simulink model "SMARTFARM_PROJ"  (R2013b)
settings: Solver=ode3  SolverMode=SingleTasking  StartTime=0.0  StopTime=10.0  RelTol=1e-3
PreLoadFcn:
  | waijung.modelPreload; % Required for working with Waijung Blockset. Do not remove.
undefined symbols (not defined in the file): HSEOSC, Link, LQFP176, ST, STM32F417IG
libraries: stm32f4_io_lib x6, stm32f4_adc_lib x1, stm32f4_device_config_lib x1
(part 2 of 2)

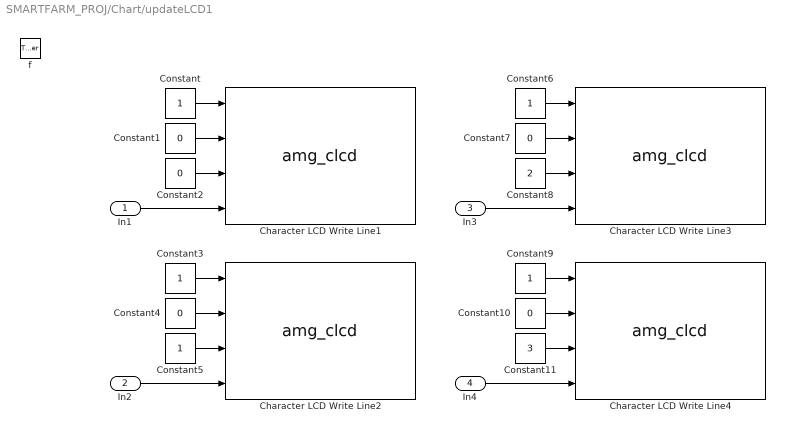
== system SMARTFARM_PROJ/Chart/updateLCD1 ==
  In1 : Inport  OutDataTypeStr=uint8  PortDimensions=[1 16]
  In2 : Inport  Port=2  OutDataTypeStr=uint8  PortDimensions=[1 16]
  In3 : Inport  Port=3  OutDataTypeStr=uint8  PortDimensions=[1 16]
  In4 : Inport  Port=4  OutDataTypeStr=uint8  PortDimensions=[1 16]
  f : TriggerPort  TriggerType=function-call
      settings: CopyFcn=Stateflow.SLINSF.SimulinkMan.removeBlockPreDeleteFcn  PreDeleteFcn=Stateflow.SLINSF.SimulinkMan.unsafePredeleteFcn
  Character LCD Write Line1 : S-Function  FunctionName=amg_clcd  Parameters=module,configuration,inputtypearray,outputtypearray,confstr,sampletime,sampletimestr,blockid  EnableBusSupport=off  mask(amg_clcd){configuration=Transaction, module=1, model=amg CLCD Std, interface=4-bits, linecount=4, columncount=20, gpiotype=Push-pull, controlport=E, control_rs=15, control_rw=13, control_en=11, dataport=A, data0=7, data1=5, data2=3, data3=1, usestringbuffer=off, stringbuffer=<empty>, varname=, inputtypearray=[4 -1 -1 -1 -1], outputtypearray=[0], confstr=["4","4","20","PP","E","15","11","13","","A","","","","","7","5","3","1","0","","1","0","0","0","1","0","0","0","0","stm32f4"], sampletime=-1, sampletimestr=-1, blockid=ChartupdateLCD1CharacterLCDWriteLine1}
      mask prompts: model "LCD model:"; linecount "Number of lines:"; columncount "Number of columns:"; gpiotype "GPIO Output type:"; controlport "GPIO control port:"; control_rs "GPIO control pin, RS:"; control_rw "GPIO control pin, RW:"; control_en "GPIO control pin, EN:"; dataport "GPIO data D[7:4] port"; data0 "GPIO data pin, D4:"; data1 "GPIO data pin, D5:"; data2 "GPIO data pin, D6:"; data3 "GPIO data pin, D7:"; usestringbuffer "Use string buffer"; stringbuffer "String buffer"; varname "Variable name"; inputtypearray "Input type array"; outputtypearray "Output type array"; confstr "Configuration string"; sampletime "Sample time (sec)"; sampletimestr "Compiled sample time (sec) in string"
      mask help:
      | Note for cmd:
      | 1 - Clear specified LCD line display before write data to LCD.
      | Otherwise (e.g. 0) - Write data without clearing LCD Line.
      |
      | Position:
      | x = 0, First Character (from left to right)
      | y = 0, Top Line
      mask init:
      | amg_clcd_callback('init');
      mask Help: web(fullfile(waijungdocroot,'amg_clcd_write.htm'), '-browser')
      mask TypeOptions configuration: Setup | Transaction
      mask Callback configuration: amg_clcd_callback('configuration');
      mask TypeOptions module: 1 | 2 | 3 | 4
      mask TypeOptions model: amg CLCD Std
      mask TypeOptions interface: 4-bits
      mask TypeOptions gpiotype: Push-pull | Open-drain
      mask TypeOptions controlport: A | B | C | D | E | F | G | H | I
      mask TypeOptions control_rs: 0 | 1 | 2 | 3 | 4 | 5 | 6 | 7 | 8 | 9 | 10 | 11 | 12 | 13 | 14 | 15
      mask TypeOptions control_rw: 0 | 1 | 2 | 3 | 4 | 5 | 6 | 7 | 8 | 9 | 10 | 11 | 12 | 13 | 14 | 15
      mask TypeOptions control_en: 0 | 1 | 2 | 3 | 4 | 5 | 6 | 7 | 8 | 9 | 10 | 11 | 12 | 13 | 14 | 15
      mask TypeOptions dataport: A | B | C | D | E | F | G | H | I
      mask TypeOptions data0: 0 | 1 | 2 | 3 | 4 | 5 | 6 | 7 | 8 | 9 | 10 | 11 | 12 | 13 | 14 | 15
      mask TypeOptions data1: 0 | 1 | 2 | 3 | 4 | 5 | 6 | 7 | 8 | 9 | 10 | 11 | 12 | 13 | 14 | 15
      mask TypeOptions data2: 0 | 1 | 2 | 3 | 4 | 5 | 6 | 7 | 8 | 9 | 10 | 11 | 12 | 13 | 14 | 15
      mask TypeOptions data3: 0 | 1 | 2 | 3 | 4 | 5 | 6 | 7 | 8 | 9 | 10 | 11 | 12 | 13 | 14 | 15
      mask Callback usestringbuffer: amg_clcd_callback('usestringbuffer');
      mask TypeOptions stringbuffer: <empty>
      mask Callback varname: amg_clcd_callback('varname');
      mask Callback confstr: amg_clcd_callback('confstr');
      mask Callback sampletime: amg_clcd_callback('sampletime');
      mask Callback sampletimestr: amg_clcd_callback('sampletimestr');
      mask Callback blockid: amg_clcd_callback('blockid');
      mask Display: text(0.5, 0.5, 'Module: CLCD1 (Write)\nTs (sec): -1','ver','middle','hor','center');port_label('input', 1,'cmd');port_label('input', 2,'xpos');port_label('input', 3,'ypos');port_label('input', 4,'str');
  Character LCD Write Line2 : S-Function  FunctionName=amg_clcd  Parameters=module,configuration,inputtypearray,outputtypearray,confstr,sampletime,sampletimestr,blockid  EnableBusSupport=off  mask(amg_clcd){configuration=Transaction, module=1, model=amg CLCD Std, interface=4-bits, linecount=4, columncount=20, gpiotype=Push-pull, controlport=E, control_rs=15, control_rw=13, control_en=11, dataport=A, data0=7, data1=5, data2=3, data3=1, usestringbuffer=off, stringbuffer=<empty>, varname=, inputtypearray=[4 -1 -1 -1 -1], outputtypearray=[0], confstr=["4","4","20","PP","E","15","11","13","","A","","","","","7","5","3","1","0","","1","0","0","0","1","0","0","0","0","stm32f4"], sampletime=-1, sampletimestr=-1, blockid=ChartupdateLCD1CharacterLCDWriteLine2}
      mask prompts: model "LCD model:"; linecount "Number of lines:"; columncount "Number of columns:"; gpiotype "GPIO Output type:"; controlport "GPIO control port:"; control_rs "GPIO control pin, RS:"; control_rw "GPIO control pin, RW:"; control_en "GPIO control pin, EN:"; dataport "GPIO data D[7:4] port"; data0 "GPIO data pin, D4:"; data1 "GPIO data pin, D5:"; data2 "GPIO data pin, D6:"; data3 "GPIO data pin, D7:"; usestringbuffer "Use string buffer"; stringbuffer "String buffer"; varname "Variable name"; inputtypearray "Input type array"; outputtypearray "Output type array"; confstr "Configuration string"; sampletime "Sample time (sec)"; sampletimestr "Compiled sample time (sec) in string"
      mask help:
      | Note for cmd:
      | 1 - Clear specified LCD line display before write data to LCD.
      | Otherwise (e.g. 0) - Write data without clearing LCD Line.
      |
      | Position:
      | x = 0, First Character (from left to right)
      | y = 0, Top Line
      mask init:
      | amg_clcd_callback('init');
      mask Help: web(fullfile(waijungdocroot,'amg_clcd_write.htm'), '-browser')
      mask TypeOptions configuration: Setup | Transaction
      mask Callback configuration: amg_clcd_callback('configuration');
      mask TypeOptions module: 1 | 2 | 3 | 4
      mask TypeOptions model: amg CLCD Std
      mask TypeOptions interface: 4-bits
      mask TypeOptions gpiotype: Push-pull | Open-drain
      mask TypeOptions controlport: A | B | C | D | E | F | G | H | I
      mask TypeOptions control_rs: 0 | 1 | 2 | 3 | 4 | 5 | 6 | 7 | 8 | 9 | 10 | 11 | 12 | 13 | 14 | 15
      mask TypeOptions control_rw: 0 | 1 | 2 | 3 | 4 | 5 | 6 | 7 | 8 | 9 | 10 | 11 | 12 | 13 | 14 | 15
      mask TypeOptions control_en: 0 | 1 | 2 | 3 | 4 | 5 | 6 | 7 | 8 | 9 | 10 | 11 | 12 | 13 | 14 | 15
      mask TypeOptions dataport: A | B | C | D | E | F | G | H | I
      mask TypeOptions data0: 0 | 1 | 2 | 3 | 4 | 5 | 6 | 7 | 8 | 9 | 10 | 11 | 12 | 13 | 14 | 15
      mask TypeOptions data1: 0 | 1 | 2 | 3 | 4 | 5 | 6 | 7 | 8 | 9 | 10 | 11 | 12 | 13 | 14 | 15
      mask TypeOptions data2: 0 | 1 | 2 | 3 | 4 | 5 | 6 | 7 | 8 | 9 | 10 | 11 | 12 | 13 | 14 | 15
      mask TypeOptions data3: 0 | 1 | 2 | 3 | 4 | 5 | 6 | 7 | 8 | 9 | 10 | 11 | 12 | 13 | 14 | 15
      mask Callback usestringbuffer: amg_clcd_callback('usestringbuffer');
      mask TypeOptions stringbuffer: <empty>
      mask Callback varname: amg_clcd_callback('varname');
      mask Callback confstr: amg_clcd_callback('confstr');
      mask Callback sampletime: amg_clcd_callback('sampletime');
      mask Callback sampletimestr: amg_clcd_callback('sampletimestr');
      mask Callback blockid: amg_clcd_callback('blockid');
      mask Display: text(0.5, 0.5, 'Module: CLCD1 (Write)\nTs (sec): -1','ver','middle','hor','center');port_label('input', 1,'cmd');port_label('input', 2,'xpos');port_label('input', 3,'ypos');port_label('input', 4,'str');
  Character LCD Write Line3 : S-Function  FunctionName=amg_clcd  Parameters=module,configuration,inputtypearray,outputtypearray,confstr,sampletime,sampletimestr,blockid  EnableBusSupport=off  mask(amg_clcd){configuration=Transaction, module=1, model=amg CLCD Std, interface=4-bits, linecount=4, columncount=20, gpiotype=Push-pull, controlport=E, control_rs=15, control_rw=13, control_en=11, dataport=A, data0=7, data1=5, data2=3, data3=1, usestringbuffer=off, stringbuffer=<empty>, varname=, inputtypearray=[4 -1 -1 -1 -1], outputtypearray=[0], confstr=["4","4","20","PP","E","15","11","13","","A","","","","","7","5","3","1","0","","1","0","0","0","1","0","0","0","0","stm32f4"], sampletime=-1, sampletimestr=-1, blockid=ChartupdateLCD1CharacterLCDWriteLine3}
      mask prompts: model "LCD model:"; linecount "Number of lines:"; columncount "Number of columns:"; gpiotype "GPIO Output type:"; controlport "GPIO control port:"; control_rs "GPIO control pin, RS:"; control_rw "GPIO control pin, RW:"; control_en "GPIO control pin, EN:"; dataport "GPIO data D[7:4] port"; data0 "GPIO data pin, D4:"; data1 "GPIO data pin, D5:"; data2 "GPIO data pin, D6:"; data3 "GPIO data pin, D7:"; usestringbuffer "Use string buffer"; stringbuffer "String buffer"; varname "Variable name"; inputtypearray "Input type array"; outputtypearray "Output type array"; confstr "Configuration string"; sampletime "Sample time (sec)"; sampletimestr "Compiled sample time (sec) in string"
      mask help:
      | Note for cmd:
      | 1 - Clear specified LCD line display before write data to LCD.
      | Otherwise (e.g. 0) - Write data without clearing LCD Line.
      |
      | Position:
      | x = 0, First Character (from left to right)
      | y = 0, Top Line
      mask init:
      | amg_clcd_callback('init');
      mask Help: web(fullfile(waijungdocroot,'amg_clcd_write.htm'), '-browser')
      mask TypeOptions configuration: Setup | Transaction
      mask Callback configuration: amg_clcd_callback('configuration');
      mask TypeOptions module: 1 | 2 | 3 | 4
      mask TypeOptions model: amg CLCD Std
      mask TypeOptions interface: 4-bits
      mask TypeOptions gpiotype: Push-pull | Open-drain
      mask TypeOptions controlport: A | B | C | D | E | F | G | H | I
      mask TypeOptions control_rs: 0 | 1 | 2 | 3 | 4 | 5 | 6 | 7 | 8 | 9 | 10 | 11 | 12 | 13 | 14 | 15
      mask TypeOptions control_rw: 0 | 1 | 2 | 3 | 4 | 5 | 6 | 7 | 8 | 9 | 10 | 11 | 12 | 13 | 14 | 15
      mask TypeOptions control_en: 0 | 1 | 2 | 3 | 4 | 5 | 6 | 7 | 8 | 9 | 10 | 11 | 12 | 13 | 14 | 15
      mask TypeOptions dataport: A | B | C | D | E | F | G | H | I
      mask TypeOptions data0: 0 | 1 | 2 | 3 | 4 | 5 | 6 | 7 | 8 | 9 | 10 | 11 | 12 | 13 | 14 | 15
      mask TypeOptions data1: 0 | 1 | 2 | 3 | 4 | 5 | 6 | 7 | 8 | 9 | 10 | 11 | 12 | 13 | 14 | 15
      mask TypeOptions data2: 0 | 1 | 2 | 3 | 4 | 5 | 6 | 7 | 8 | 9 | 10 | 11 | 12 | 13 | 14 | 15
      mask TypeOptions data3: 0 | 1 | 2 | 3 | 4 | 5 | 6 | 7 | 8 | 9 | 10 | 11 | 12 | 13 | 14 | 15
      mask Callback usestringbuffer: amg_clcd_callback('usestringbuffer');
      mask TypeOptions stringbuffer: <empty>
      mask Callback varname: amg_clcd_callback('varname');
      mask Callback confstr: amg_clcd_callback('confstr');
      mask Callback sampletime: amg_clcd_callback('sampletime');
      mask Callback sampletimestr: amg_clcd_callback('sampletimestr');
      mask Callback blockid: amg_clcd_callback('blockid');
      mask Display: text(0.5, 0.5, 'Module: CLCD1 (Write)\nTs (sec): -1','ver','middle','hor','center');port_label('input', 1,'cmd');port_label('input', 2,'xpos');port_label('input', 3,'ypos');port_label('input', 4,'str');
  Character LCD Write Line4 : S-Function  FunctionName=amg_clcd  Parameters=module,configuration,inputtypearray,outputtypearray,confstr,sampletime,sampletimestr,blockid  EnableBusSupport=off  mask(amg_clcd){configuration=Transaction, module=1, model=amg CLCD Std, interface=4-bits, linecount=4, columncount=20, gpiotype=Push-pull, controlport=E, control_rs=15, control_rw=13, control_en=11, dataport=A, data0=7, data1=5, data2=3, data3=1, usestringbuffer=off, stringbuffer=<empty>, varname=, inputtypearray=[4 -1 -1 -1 -1], outputtypearray=[0], confstr=["4","4","20","PP","E","15","11","13","","A","","","","","7","5","3","1","0","","1","0","0","0","1","0","0","0","0","stm32f4"], sampletime=-1, sampletimestr=-1, blockid=ChartupdateLCD1CharacterLCDWriteLine4}
      mask prompts: model "LCD model:"; linecount "Number of lines:"; columncount "Number of columns:"; gpiotype "GPIO Output type:"; controlport "GPIO control port:"; control_rs "GPIO control pin, RS:"; control_rw "GPIO control pin, RW:"; control_en "GPIO control pin, EN:"; dataport "GPIO data D[7:4] port"; data0 "GPIO data pin, D4:"; data1 "GPIO data pin, D5:"; data2 "GPIO data pin, D6:"; data3 "GPIO data pin, D7:"; usestringbuffer "Use string buffer"; stringbuffer "String buffer"; varname "Variable name"; inputtypearray "Input type array"; outputtypearray "Output type array"; confstr "Configuration string"; sampletime "Sample time (sec)"; sampletimestr "Compiled sample time (sec) in string"
      mask help:
      | Note for cmd:
      | 1 - Clear specified LCD line display before write data to LCD.
      | Otherwise (e.g. 0) - Write data without clearing LCD Line.
      |
      | Position:
      | x = 0, First Character (from left to right)
      | y = 0, Top Line
      mask init:
      | amg_clcd_callback('init');
      mask Help: web(fullfile(waijungdocroot,'amg_clcd_write.htm'), '-browser')
      mask TypeOptions configuration: Setup | Transaction
      mask Callback configuration: amg_clcd_callback('configuration');
      mask TypeOptions module: 1 | 2 | 3 | 4
      mask TypeOptions model: amg CLCD Std
      mask TypeOptions interface: 4-bits
      mask TypeOptions gpiotype: Push-pull | Open-drain
      mask TypeOptions controlport: A | B | C | D | E | F | G | H | I
      mask TypeOptions control_rs: 0 | 1 | 2 | 3 | 4 | 5 | 6 | 7 | 8 | 9 | 10 | 11 | 12 | 13 | 14 | 15
      mask TypeOptions control_rw: 0 | 1 | 2 | 3 | 4 | 5 | 6 | 7 | 8 | 9 | 10 | 11 | 12 | 13 | 14 | 15
      mask TypeOptions control_en: 0 | 1 | 2 | 3 | 4 | 5 | 6 | 7 | 8 | 9 | 10 | 11 | 12 | 13 | 14 | 15
      mask TypeOptions dataport: A | B | C | D | E | F | G | H | I
      mask TypeOptions data0: 0 | 1 | 2 | 3 | 4 | 5 | 6 | 7 | 8 | 9 | 10 | 11 | 12 | 13 | 14 | 15
      mask TypeOptions data1: 0 | 1 | 2 | 3 | 4 | 5 | 6 | 7 | 8 | 9 | 10 | 11 | 12 | 13 | 14 | 15
      mask TypeOptions data2: 0 | 1 | 2 | 3 | 4 | 5 | 6 | 7 | 8 | 9 | 10 | 11 | 12 | 13 | 14 | 15
      mask TypeOptions data3: 0 | 1 | 2 | 3 | 4 | 5 | 6 | 7 | 8 | 9 | 10 | 11 | 12 | 13 | 14 | 15
      mask Callback usestringbuffer: amg_clcd_callback('usestringbuffer');
      mask TypeOptions stringbuffer: <empty>
      mask Callback varname: amg_clcd_callback('varname');
      mask Callback confstr: amg_clcd_callback('confstr');
      mask Callback sampletime: amg_clcd_callback('sampletime');
      mask Callback sampletimestr: amg_clcd_callback('sampletimestr');
      mask Callback blockid: amg_clcd_callback('blockid');
      mask Display: text(0.5, 0.5, 'Module: CLCD1 (Write)\nTs (sec): -1','ver','middle','hor','center');port_label('input', 1,'cmd');port_label('input', 2,'xpos');port_label('input', 3,'ypos');port_label('input', 4,'str');
  Constant{,3,5..6,9} (5 alike) : Constant
  Constant{1..2,4,7,10} (5 alike) : Constant  Value=0
  Constant11 : Constant  Value=3
  Constant8 : Constant  Value=2
  wires:
  In1/1 -> Character LCD Write Line1/4
  Constant/1 -> Character LCD Write Line1/1
  Constant1/1 -> Character LCD Write Line1/2
  Constant2/1 -> Character LCD Write Line1/3
  In2/1 -> Character LCD Write Line2/4
  Constant3/1 -> Character LCD Write Line2/1
  Constant4/1 -> Character LCD Write Line2/2
  Constant5/1 -> Character LCD Write Line2/3
  In3/1 -> Character LCD Write Line3/4
  Constant6/1 -> Character LCD Write Line3/1
  Constant7/1 -> Character LCD Write Line3/2
  Constant8/1 -> Character LCD Write Line3/3
  In4/1 -> Character LCD Write Line4/4
  Constant9/1 -> Character LCD Write Line4/1
  Constant10/1 -> Character LCD Write Line4/2
  Constant11/1 -> Character LCD Write Line4/3

== stateflow chart SMARTFARM_PROJ/Chart ==
  state Initialization
  state NormalOperation
    state CheckKeyPress [parallel]
      settings: executionOrder=2
      state NoKeyPressed
        en: data = 0;
      state UpKeyPressed
        en: data = 1;
        state Short
        (default) -> NormalOperation.CheckKeyPress.UpKeyPressed.Short : {UP_KEY_PRESSED;}
      state DownKeyPressed
        en: data = 1;
        state Short
        state Long
        state wait
        (default) -> NormalOperation.CheckKeyPress.DownKeyPressed.Short : {DOWN_KEY_PRESSED;}
        NormalOperation.CheckKeyPress.DownKeyPressed.Short -> NormalOperation.CheckKeyPress.DownKeyPressed.Long : after(1,sec)
        NormalOperation.CheckKeyPress.DownKeyPressed.Long -> wait
      state OkKeyPressed
        en: data = 1;
        state Short
        state Long
        (default) -> NormalOperation.CheckKeyPress.OkKeyPressed.Short : {OK_KEY_PRESSED;}
        NormalOperation.CheckKeyPress.OkKeyPressed.Short -> NormalOperation.CheckKeyPress.OkKeyPressed.Long : after(1,sec)
      (default) -> NoKeyPressed
      NoKeyPressed -> UpKeyPressed [order 1] : [up_key == 1]
      UpKeyPressed -> NoKeyPressed : [up_key == 0]
      NoKeyPressed -> DownKeyPressed [order 2] : [down_key == 1]
      DownKeyPressed -> NoKeyPressed : [down_key == 0]
      NoKeyPressed -> OkKeyPressed [order 3] : [ok_key == 1]
      OkKeyPressed -> NoKeyPressed : [ok_key == 0]
    state MenuDisplay [parallel]
      settings: executionOrder=1
      state Screen3
        en: lcd_line1 = setLcdLine1(4);
        en: updateSol();
        en: updateFerA();
        en: updateFerB();
        en: updateLCD1(lcd_line1,lcd_line2,lcd_line3,lcd_line4);
      state Screen2
        en: lcd_line1 = setLcdLine1(2);
        en: lcd_line2 = setLcdLine2(2);
        en: lcd_line3 = setLcdLine3(5);
        en: updateAuto();
        en: updateLCD1(lcd_line1,lcd_line2,lcd_line3,lcd_line4);
      state Screen1
        en: lcd_line1 = setLcdLine1(1);
        en: lcd_line2 = setLcdLine2(1);
        en: lcd_line3 = setLcdLine3(1);
        en: lcd_line4 = setLcdLine4(1);
        en: updateLCD1(lcd_line1,lcd_line2,lcd_line3,lcd_line4);
      state Screen21
        en: lcd_line1 = setLcdLine1(2);
        en: lcd_line2 = setLcdLine2(10);
        en: lcd_line3 = setLcdLine3(4);
        en: updateAuto();
        en: updateLCD1(lcd_line1,lcd_line2,lcd_line3,lcd_line4);
      state Screen23
        en: lcd_line1 = setLcdLine1(4);
        en: updateFerA2();
        en: updateFerB3();
        en: updateMoist();
        en: updateLCD1(lcd_line1,lcd_line2,lcd_line3,lcd_line4);
      state Screen4
        en: lcd_line1 = setLcdLine1(4);
        en: totalDate();
        en: startDate();
        en: lcd_line4 = setLcdLine4(0);
        en: updateLCD1(lcd_line1,lcd_line2,lcd_line3,lcd_line4);
      state Screen22
        en: lcd_line1 = setLcdLine1(2);
        en: lcd_line2 = setLcdLine2(4);
        en: lcd_line3 = setLcdLine3(3);
        en: updateAuto();
        en: updateLCD1(lcd_line1,lcd_line2,lcd_line3,lcd_line4);
      state Screen5
        en: lcd_line1 = setLcdLine1(6);
        en: upTIme();
        en: lcd_line3 = setLcdLine3(0);
        en: lcd_line4 = setLcdLine4(0);
        en: updateLCD1(lcd_line1,lcd_line2,lcd_line3,lcd_line4);
      Screen3 -> Screen3 [order 2] : after(1.5,sec)
      Screen2 -> Screen2 [order 3] : after(1.5,sec)
      (default) -> Screen1
      Screen2 -> Screen3 [order 2] : OK_KEY_PRESSED
      Screen3 -> Screen2 [order 1] : [in(CheckKeyPress.DownKeyPressed.Long)]
      Screen1 -> Screen2 : OK_KEY_PRESSED
      Screen23 -> Screen3 [order 3] : UP_KEY_PRESSED
      Screen3 -> Screen23 [order 3] : DOWN_KEY_PRESSED
      Screen23 -> Screen2 [order 1] : [in(CheckKeyPress.DownKeyPressed.Long)]
      Screen2 -> Screen21 [order 1] : DOWN_KEY_PRESSED
      Screen21 -> Screen2 [order 3] : UP_KEY_PRESSED
      Screen23 -> Screen23 [order 2] : after(1.5,sec)
      Screen21 -> Screen22 [order 1] : DOWN_KEY_PRESSED
      Screen22 -> Screen21 [order 1] : UP_KEY_PRESSED
      Screen4 -> Screen21 [order 1] : [in(CheckKeyPress.DownKeyPressed.Long)]
      Screen21 -> Screen4 [order 2] : OK_KEY_PRESSED
      Screen4 -> Screen4 [order 2] : after(1.5,sec)
      Screen22 -> Screen5 [order 2] : OK_KEY_PRESSED
      Screen5 -> Screen22 : [in(CheckKeyPress.DownKeyPressed.Long)]
  state updateLCD1(In1,In2,In3,In4) [function]
  (default) -> Initialization
  Initialization -> NormalOperation
  data: option function_input double; outstr function_output uint8 size=[1 16]; option function_input double; outstr function_output uint8 size=[1 16]; option function_input double; outstr function_output uint8 size=[1 16]; option function_input double; outstr function_output uint8 size=[1 16]; In1 function_input uint8 size=[1 16]; In2 function_input uint8 size=[1 16]; In3 function_input uint8 size=[1 16]; In4 function_input uint8 size=[1 16]; ok_key input; up_key input; down_key input; data output double =0; lcd_line1 local uint8 size=[1 16]; lcd_line2 local uint8 size=[1 16]; lcd_line3 local uint8 size=[1 16]; lcd_line4 local uint8 size=[1 16]; FERT_A_VALUE input int32; FERT_B_VALUE input int32; SOL_VALVE input int32; AUTO input int32; totalDate1 input int32; startDate1 input int32; moistVal input; hourVal input; minVal input; secVal input
  events: triger input RISING_EDGE_EVENT; UP_KEY_PRESSED local FUNCTION_CALL_EVENT; OK_KEY_PRESSED local FUNCTION_CALL_EVENT; DOWN_KEY_PRESSED local FUNCTION_CALL_EVENT; DOWN_KEY_HOLD local FUNCTION_CALL_EVENT
  function outstr = setLcdLine1(option):
    | function outstr = setLcdLine1(option)
    | 
    | switch option
    |     case 0             %0123456789ABCDEF
    |         outstr = uint8('                ');
    |     case 1  
    |         outstr = uint8('   SMART FARM   ');
    |     case 2 
    |         outstr = uint8('  *Main Menu*   ');
    |     case 3
    |         outstr = uint8('   *  RUN   *   ');
    |     case 4
    |         outstr = uint8('  * MONITOR *   ');
    |     case 5
    |         outstr = uint8(' * SET Alarm  * ');
    |     case 6
    |         outstr = uint8('*     TIME     *');
    |     case 7
    |         outstr = uint8('  *  MONITOR *  ');
    |     otherwise
    |         outstr = uint8('                ');
    | end
  function outstr = setLcdLine2(option):
    | function outstr = setLcdLine2(option)
    | 
    | switch option
    |     case 0             %0123456789ABCDEF
    |         outstr = uint8('                ');
    |     case 1  
    |         outstr = uint8('By Pathompong C.');
    |     case 2 
    |         outstr = uint8('>MONITOR        ');
    |     case 3
    |         outstr = uint8(' MONITOR        ');
    |     case 4
    |         outstr = uint8(' DATE           ');
    |     case 5
    |         outstr = uint8('>Setpoint=XX Deg');
    |     case 6
    |         outstr = uint8('>HighAlarm=XX % '); 
    |     case 7
    |         outstr = uint8(' HighAlarm=XX % ');
    |     case 8
    |         outstr = uint8('Time: XX :XX :XX');
    |     case 9
    |         outstr = uint8('>MONITOR        ');
    |     case 10
    |         outstr = uint8(' MONITOR        ');
    |     otherwise
    |         outstr = uint8('                ');
    | end
  function updateFerA:
    | function updateFerA
    | if (FERT_A_VALUE == 1)
    |                                                 %'123456789ABCDEFG'
    |     coder.ceval('sprintf',coder.ref(lcd_line3), ['FerA: ON        ']);
    | else
    |     coder.ceval('sprintf',coder.ref(lcd_line3), ['FerA: OFF       ']);
    | end
    | 
    | 
    | 
    | 
    | %
  function updateAuto:
    | function updateAuto
    | if (AUTO == 1)
    |                                                 %'123456789ABCDEFG'
    |     coder.ceval('sprintf',coder.ref(lcd_line4), ['AUTO: ON        ']);
    | else
    |     coder.ceval('sprintf',coder.ref(lcd_line4), ['AUTO: OFF       ']);
    | end
  function updateFerB:
    | function updateFerB
    | if (FERT_B_VALUE == 1)
    |                                                 %'123456789ABCDEFG'
    |     coder.ceval('sprintf',coder.ref(lcd_line4), ['FerB: ON        ']);
    | else
    |     coder.ceval('sprintf',coder.ref(lcd_line4), ['FerB: OFF       ']);
    | end
  function startDate:
    | function startDate
    |                                             %'123456789ABCDEFG
    | coder.ceval('sprintf',coder.ref(lcd_line3), ['StartDate: %d   '], startDate1);
  function updateSol:
    | function updateSol
    | if (SOL_VALVE == 1)
    |                                                 %'123456789ABCDEFG'
    |     coder.ceval('sprintf',coder.ref(lcd_line2), ['Sol Val: ON     ']);
    | else
    |     coder.ceval('sprintf',coder.ref(lcd_line2), ['Sol Val: OFF    ']);
    | end
  function totalDate:
    | function totalDate
    |                                             %'123456789ABCDEFG
    | coder.ceval('sprintf',coder.ref(lcd_line2), ['TotalDate: %d   '], totalDate1);
  function updateFerA2:
    | function updateFerA2
    | if (FERT_A_VALUE == 1)
    |                                                 %'123456789ABCDEFG'
    |     coder.ceval('sprintf',coder.ref(lcd_line2), ['FerA: ON        ']);
    | else
    |     coder.ceval('sprintf',coder.ref(lcd_line2), ['FerA: OFF       ']);
    | end
    | 
    | 
    | 
    | 
    | %
  function updateMoist:
    | function updateMoist
    |                                             %'123456789ABCDEFG'
    | coder.ceval('sprintf',coder.ref(lcd_line4), ['Moisture: %.2f    '], moistVal);
  function upTIme:
    | function upTIme
    |                                             %'123456789ABCDEFG'
    | coder.ceval('sprintf',coder.ref(lcd_line2), ['Time: %d :%d :%d'], hourVal, minVal, secVal);
  function updateFerB3:
    | function updateFerB3
    | if (FERT_B_VALUE == 1)
    |                                                 %'123456789ABCDEFG'
    |     coder.ceval('sprintf',coder.ref(lcd_line3), ['FerB: ON        ']);
    | else
    |     coder.ceval('sprintf',coder.ref(lcd_line3), ['FerB: OFF       ']);
    | end
  function outstr = setLcdLine3(option):
    | function outstr = setLcdLine3(option)
    | 
    | switch option
    |     case 0             %0123456789ABCDEF
    |         outstr = uint8('                ');
    |     case 1  
    |         outstr = uint8('  MICHELLE M.   ');
    |     case 2 
    |         outstr = uint8(' TIME           ');
    |     case 3
    |         outstr = uint8('>TIME           ');
    |     case 4
    |         outstr = uint8('>DATE           ');
    |     case 5
    |         outstr = uint8(' DATE           ');
    |     case 6
    |         outstr = uint8('Fer-A=OFF       ');
    |     case 7
    |         outstr = uint8('Moisture:XX.X % ');
    |     
    |     otherwise
    |         outstr = uint8('                ');
    | end
  function outstr = setLcdLine4(option):
    | function outstr = setLcdLine4(option)
    | 
    | switch option
    |     case 0             %0123456789ABCDEF
    |         outstr = uint8('                ');
    |     case 1  
    |         outstr = uint8('      ABAC      ');
    |     case 2 
    |         outstr = uint8(' SET Alarm      ');
    |     case 3
    |         outstr = uint8('>SET Alarm      ');
    |     case 4
    |         outstr = uint8('ER: ZZ Deg      ');
    |     case 7
    |         outstr = uint8(' MANUAL         ');
    |     case 8
    |         outstr = uint8('Fer-B = OFF     ');
    |     otherwise
    |         outstr = uint8('                ');
    | end
